simulink model "sensor_fusion_1"  (R2022b)
settings: Solver=FixedStepAuto  StartTime=0.0  StopTime=142  RelTol=1e-3  EnableMultiTasking=on
values from neighbouring files (symbols this model uses):
  A = [1.06559801427  0.0478097134081  -0.0142426631232; 0.0478097134081  0.959164863261  -0.0359507847494; -0.0142426631232  -0.0359507847494  0.982079248423]    [run1.mat]    (also in run1_wscan.mat; run2.mat; run2_wscan.mat; run3_wscan.mat)
  b = [2.14306210308 15.720848335 -0.863601368467]    [run1.mat]    (also in run1_wscan.mat; run2.mat; run2_wscan.mat; run3_wscan.mat)
  lut_in_model = [0.613658288305 4.0918386519 6.33532627088 8.02783554654 9.39128126795 10.3149653152 11.0684466084 11.9394591465 12.6234642167 13.2815233141 13.7919727262 14.1169774697 ... (18 elements, 1x18)]    [lut1.mat]    (also in lut2.mat = [2.20352000565 5.28649692724 7.42737645164 9.16368787483 10.; lut3.mat = [3.87191743285 4.36123645733 5.94318349981 7.0907146991 9.12; lut4.mat = [4.07430286502 6.74924870692 8.79421351968 10.2475792888 11.; run7_wscan.mat = [4.07430286502 6.74924870692 8.79421351968 10.2475792888 11.)
  lut_out_model = [4.36363636364 5.45454545455 6.54545454545 7.63636363636 8.72727272727 9.81818181818 10.9090909091 12 13.0909090909 14.1818181818 15.2727272727 16.3636363636 ... (18 elements, 1x18)]    [lut1.mat]    (also in lut2.mat; lut3.mat = [4.14545454545 4.36363636364 4.90909090909 5.45454545455 6.5; lut4.mat; run7_wscan.mat)
undefined symbols (not defined in the file or in its folder): ODR
libraries: raspberrypiBasiclib x6, simulink x4, raspberrypiIMUsensorslib x2, robotmobilelib x1, dspsigops x1
settings Model: Creator=sjohnson  LastModifiedBy=sjohnson
settings SolverCC: PositivePriorityOrder=on
settings OptimizationCC: EnhancedBackFolding=on  PassReuseOutputArgsAs=Individual arguments  ZeroExternalMemoryAtStartup=off  ZeroInternalMemoryAtStartup=off  MaxStackSize=64  OptimizeBlockOrder=speed  DifferentSizesBufferReuse=on  OptimizationCustomize=off  EfficientTunableParamExpr=on
settings DebuggingCC: ParameterTunabilityLossMsg=error
settings HardwareCC: ProdBitPerPointer=32  ProdBitPerSizeT=32  ProdBitPerPtrDiffT=32  ProdLargestAtomicInteger=Long  ProdLargestAtomicFloat=Double  ProdWordSize=32  ProdLongLongMode=on  ProdHWDeviceType=ARM Compatible->ARM Cortex  UseEmbeddedCoderFeatures=off  UseSimulinkCoderFeatures=off
settings RTWCC: Description=Embedded Coder  SystemTargetFile=ert.tlc  HardwareBoard=Raspberry Pi  TLCOptions="-aInlineSetEventsForThisBaseRateFcn=TLC_FALSE -aSuppressMultiTaskScheduler=TLC_FALSE  -aRateBasedStepFcn=0"  TemplateMakefile=ert_default_tmf  Toolchain=GNU GCC Embedded Linux  BuildConfiguration=Faster Runs
settings CodeAppCC: ForceParamTrailComments=on  IgnoreCustomStorageClasses=off  OperatorAnnotations=on  SimulinkDataObjDesc=on  SFDataObjDesc=on  InsertBlockDesc=on
settings ERTTargetCC: SupportNonInlinedSFcns=on  SupportVariableSizeSignals=on  ExtModeTransport=2  ExtModeStaticAlloc=on  ExtModeMexFile=ext_xcp  ExtModeIntrfLevel=Level2 - Open

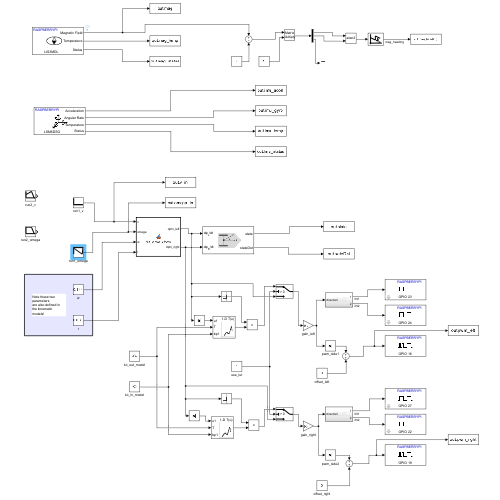
[thumbnail: Simulink's stored preview of the top-level diagram]
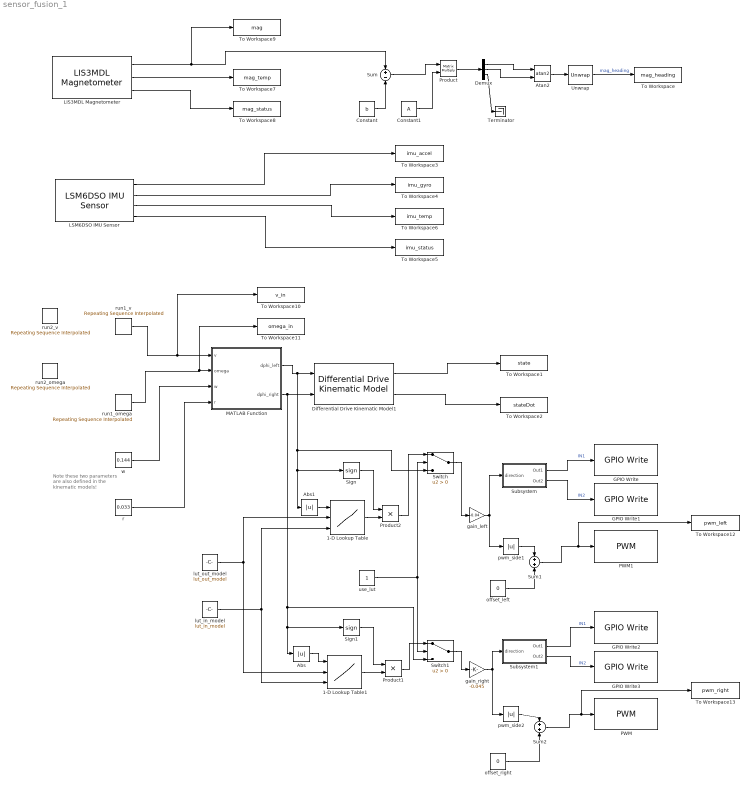
== system sensor_fusion_1 ==
  note: Note these two parameters
      | are also defined in the kinematic
      | models!
  1-D Lookup Table : Lookup_n-D  NumberOfTableDimensions=1  BreakpointsForDimension1Source=Input port  BreakpointsForDimension1=[-5:5]  IndexSearchMethod=Linear search  TableSource=Input port  Table=tanh([-5:5])  InterpMethod=Cubic spline  InternalRulePriority=Speed  RndMeth=Simplest
      settings: InputPortMap=u0,p221,p5
  1-D Lookup Table1 : Lookup_n-D  NumberOfTableDimensions=1  BreakpointsForDimension1Source=Input port  BreakpointsForDimension1=[-5:5]  IndexSearchMethod=Linear search  TableSource=Input port  Table=tanh([-5:5])  InterpMethod=Cubic spline  InternalRulePriority=Speed  RndMeth=Simplest
      settings: InputPortMap=u0,p221,p5
  Abs : Abs  SaturateOnIntegerOverflow=off
  Abs1 : Abs  SaturateOnIntegerOverflow=off
  Atan2 : Trigonometry  Operator=atan2
  Constant : Constant  Value=b
  Constant1 : Constant  Value=A
  Demux : Demux  Outputs=3
  Differential Drive Kinematic Model1 : robotmobilelib/Differential Drive Kinematic Model  VehicleInputs=Wheel Speeds  WheelRadius=.033  WheelSpeedRange=[-inf inf]  TrackWidth=0.144  InitialState=[0; 0; 0]  SimulateUsing=Interpreted execution
  GPIO Write : raspberrypiBasiclib/GPIO Write  board=Pi 4 Model B  gpio=23  direction=Output  blockPlatform=Raspberry Pi
  GPIO Write1 : raspberrypiBasiclib/GPIO Write  board=Pi 4 Model B  gpio=24  direction=Output  blockPlatform=Raspberry Pi
  GPIO Write2 : raspberrypiBasiclib/GPIO Write  board=Pi 4 Model B  gpio=27  direction=Output  blockPlatform=Raspberry Pi
  GPIO Write3 : raspberrypiBasiclib/GPIO Write  board=Pi 4 Model B  gpio=22  direction=Output  blockPlatform=Raspberry Pi
  LIS3MDL Magnetometer : raspberrypiIMUsensorslib/LIS3MDL Magnetometer  I2CModule=1  I2CAddress=0x1E  IsActiveMagnetometer=on  IsActiveTemperature=on  IsStatus=on  SampleTime=-1  MagnetometerRange=+/- 400 uT  MagnetometerODR=40 Hz
  LSM6DSO IMU Sensor : raspberrypiIMUsensorslib/LSM6DSO IMU Sensor  I2CModule=1  I2CAddress=0x6B  IsActiveAcceleration=on  IsActiveAngularRate=on  IsActiveTemperature=on  IsActiveStatus=on  IsActiveTimeStamp=off  SampleTime=-1  QueueSizeFactor=3  AccelerometerRange=+/- 2g  AccelerometerODR=52 Hz  AccelSelectCompositeFilter=No filter  AccelLPF2BW=ODR/4  AccelHPFBW=ODR/4  GyroscopeRange=1000 dps  GyroscopeODR=52 Hz  EnableGyroHPF=off  GyroHPFBW=0.016 Hz  EnableGyroLPF=off  GyroLPFBWMode=0
  MATLAB Function : MATLAB Function  TreatAsAtomicUnit=on
  PWM : raspberrypiBasiclib/PWM  board=Pi 4 Model B  Pin_=19  Frequency=40  blockPlatform=Raspberry Pi
  PWM1 : raspberrypiBasiclib/PWM  board=Pi 4 Model B  Pin_=18  Frequency=40  blockPlatform=Raspberry Pi
  Product : Product  Multiplication=Matrix(*)
  Product1 : Product
  Product2 : Product
  Sign : Signum
  Sign1 : Signum
  Subsystem : Subsystem
  Subsystem1 : Subsystem
  Sum : Sum  Inputs=+-
  Sum1 : Sum
  Sum2 : Sum
  Switch : Switch  Criteria=u2 > Threshold  SaturateOnIntegerOverflow=off  InputSameDT=off
  Switch1 : Switch  Criteria=u2 > Threshold  SaturateOnIntegerOverflow=off  InputSameDT=off
  Terminator : Terminator
  To Workspace : ToWorkspace  VariableName=mag_heading  SaveFormat=Structure With Time  SampleTime=-1
  To Workspace1 : ToWorkspace  VariableName=state  SaveFormat=Structure With Time  SampleTime=-1
  To Workspace10 : ToWorkspace  VariableName=v_in  SaveFormat=Structure With Time  SampleTime=-1
  To Workspace11 : ToWorkspace  VariableName=omega_in  SaveFormat=Structure With Time  SampleTime=-1
  To Workspace12 : ToWorkspace  VariableName=pwm_left  SaveFormat=Structure With Time  SampleTime=-1
  To Workspace13 : ToWorkspace  VariableName=pwm_right  SaveFormat=Structure With Time  SampleTime=-1
  To Workspace2 : ToWorkspace  VariableName=stateDot  SaveFormat=Structure With Time  SampleTime=-1
  To Workspace3 : ToWorkspace  VariableName=imu_accel  SaveFormat=Structure With Time  SampleTime=-1
  To Workspace4 : ToWorkspace  VariableName=imu_gyro  SaveFormat=Structure With Time  SampleTime=-1
  To Workspace5 : ToWorkspace  VariableName=imu_status  SaveFormat=Structure With Time  SampleTime=-1
  To Workspace6 : ToWorkspace  VariableName=imu_temp  SaveFormat=Structure With Time  SampleTime=-1
  To Workspace7 : ToWorkspace  VariableName=mag_temp  SaveFormat=Structure With Time  SampleTime=-1
  To Workspace8 : ToWorkspace  VariableName=mag_status  SaveFormat=Structure With Time  SampleTime=-1
  To Workspace9 : ToWorkspace  VariableName=mag  SaveFormat=Structure With Time  SampleTime=-1
  Unwrap : dspsigops/Unwrap  tol=pi  InputProcessing=Columns as channels (frame based)  running=off
  gain_left : Gain  Gain=-0.04
  gain_right : Gain  Gain=-0.045
  lut_in_model : Constant  Value=lut_in_model
  lut_out_model : Constant  Value=lut_out_model
  offset_left : Constant  Value=0
  offset_right : Constant  Value=0
  pwm_side1 : Abs  SaturateOnIntegerOverflow=off
  pwm_side2 : Abs  SaturateOnIntegerOverflow=off
  r : Constant  Value=0.033
  run1_omega : simulink/Sources/Repeating Sequence Interpolated  OutValues=-[0.5 1.0 1.5 2.0 2.5 3 3.5 4 4.5 5 5.5 6 6.5 7 0 0]  TimeValues=[0:10:140 142]  LookUpMeth=Use Input Below  tsamp=0.01  OutMin=[]  OutMax=[]  OutDataTypeStr=double  OutputDataTypeScalingMode=double  OutDataType=fixdt(0,8)  OutScaling=2^-10
  run1_v : simulink/Sources/Repeating Sequence Interpolated  OutValues=[0 0 0 0 0 0 0 0 0 0 0 0 0 0 0 0 0 0 0 0 0 0 0 0 0]  TimeValues=[0:10:230 232]  LookUpMeth=Use Input Below  tsamp=0.01  OutMin=[]  OutMax=[]  OutDataTypeStr=double  OutputDataTypeScalingMode=double  OutDataType=fixdt(0,8)  OutScaling=2^-10
  run2_omega : simulink/Sources/Repeating Sequence Interpolated  OutValues=[1 1 1 0.0 0.0]  TimeValues=[0 5 10 15 17]  LookUpMeth=Use Input Below  tsamp=0.01  OutMin=[]  OutMax=[]  OutDataTypeStr=double  OutputDataTypeScalingMode=double  OutDataType=fixdt(0,8)  OutScaling=2^-10
  run2_v : simulink/Sources/Repeating Sequence Interpolated  OutValues=[0.2 0.3 0.4 0 0]  TimeValues=[0 5 10 15 17]  LookUpMeth=Use Input Below  tsamp=0.01  OutMin=[]  OutMax=[]  OutDataTypeStr=double  OutputDataTypeScalingMode=double  OutDataType=fixdt(0,8)  OutScaling=2^-10
  use_lut : Constant
  w : Constant  Value=0.144
  wires:
  Differential Drive Kinematic Model1/1 -> To Workspace1/1
  Unwrap/1 -> To Workspace/1  "mag_heading"
  offset_right/1 -> Sum2/2
  Sum1/1 -> To Workspace12/1, PWM1/1
  pwm_side1/1 -> Sum1/1
  Sum2/1 -> To Workspace13/1, PWM/1
  MATLAB Function/2(dphi_right) -> Switch1/3, Sign1/1, Abs/1, Differential Drive Kinematic Model1/2
  Demux/1 -> Atan2/1
  Subsystem1/1(Out1) -> GPIO Write2/1  "IN1"
  Sum/1 -> Product/1
  Subsystem/1(Out1) -> GPIO Write/1  "IN1"
  Subsystem1/2(Out2) -> GPIO Write3/1  "IN2"
  offset_left/1 -> Sum1/2
  LIS3MDL Magnetometer/1 -> To Workspace9/1, Sum/1
  w/1 -> MATLAB Function/3(w)
  gain_right/1 -> pwm_side2/1, Subsystem1/1(direction)
  Atan2/1 -> Unwrap/1
  Constant/1 -> Sum/2
  run1_omega/1 -> To Workspace11/1, MATLAB Function/2(omega)
  pwm_side2/1 -> Sum2/1
  r/1 -> MATLAB Function/4(r)
  Differential Drive Kinematic Model1/2 -> To Workspace2/1
  LIS3MDL Magnetometer/3 -> To Workspace8/1
  gain_left/1 -> pwm_side1/1, Subsystem/1(direction)
  Subsystem/2(Out2) -> GPIO Write1/1  "IN2"
  MATLAB Function/1(dphi_left) -> Switch/3, Sign/1, Abs1/1, Differential Drive Kinematic Model1/1
  Demux/2 -> Atan2/2
  LIS3MDL Magnetometer/2 -> To Workspace7/1
  Constant1/1 -> Product/2
  Product/1 -> Demux/1
  LSM6DSO IMU Sensor/1 -> To Workspace3/1
  LSM6DSO IMU Sensor/4 -> To Workspace5/1
  LSM6DSO IMU Sensor/2 -> To Workspace4/1
  LSM6DSO IMU Sensor/3 -> To Workspace6/1
  Demux/3 -> Terminator/1
  run1_v/1 -> To Workspace10/1, MATLAB Function/1(v)
  lut_in_model/1 -> 1-D Lookup Table1/3, 1-D Lookup Table/3
  lut_out_model/1 -> 1-D Lookup Table1/2, 1-D Lookup Table/2
  1-D Lookup Table1/1 -> Product1/2
  Abs/1 -> 1-D Lookup Table1/1
  Abs1/1 -> 1-D Lookup Table/1
  Product1/1 -> Switch1/1
  Sign1/1 -> Product1/1
  Product2/1 -> Switch/1
  Sign/1 -> Product2/1
  1-D Lookup Table/1 -> Product2/2
  use_lut/1 -> Switch1/2, Switch/2
  Switch/1 -> gain_left/1
  Switch1/1 -> gain_right/1

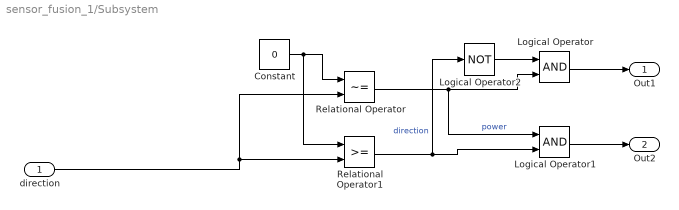
== system sensor_fusion_1/Subsystem ==
  direction : Inport
  Constant : Constant  Value=0
  Logical Operator : Logic  AllPortsSameDT=off  OutDataTypeStr=boolean
  Logical Operator1 : Logic  AllPortsSameDT=off  OutDataTypeStr=boolean
  Logical Operator2 : Logic  Operator=NOT  Inputs=1  AllPortsSameDT=off  OutDataTypeStr=boolean
  Relational Operator : RelationalOperator  Operator=~=  OutDataTypeStr=boolean  RndMeth=Simplest  InputSameDT=off
  Relational Operator1 : RelationalOperator  OutDataTypeStr=boolean  RndMeth=Simplest  InputSameDT=off
  Out1 : Outport
  Out2 : Outport  Port=2
  wires:
  Logical Operator/1 -> Out1/1
  Relational Operator1/1 -> Logical Operator2/1, Logical Operator1/2  "direction"
  Logical Operator1/1 -> Out2/1
  Logical Operator2/1 -> Logical Operator/1
  direction/1 -> Relational Operator/2, Relational Operator1/2
  Constant/1 -> Relational Operator1/1, Relational Operator/1
  Relational Operator/1 -> Logical Operator1/1, Logical Operator/2  "power"

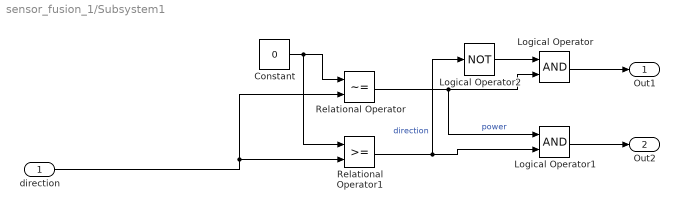
== system sensor_fusion_1/Subsystem1 ==
  direction : Inport
  Constant : Constant  Value=0
  Logical Operator : Logic  AllPortsSameDT=off  OutDataTypeStr=boolean
  Logical Operator1 : Logic  AllPortsSameDT=off  OutDataTypeStr=boolean
  Logical Operator2 : Logic  Operator=NOT  Inputs=1  AllPortsSameDT=off  OutDataTypeStr=boolean
  Relational Operator : RelationalOperator  Operator=~=  OutDataTypeStr=boolean  RndMeth=Simplest  InputSameDT=off
  Relational Operator1 : RelationalOperator  OutDataTypeStr=boolean  RndMeth=Simplest  InputSameDT=off
  Out1 : Outport
  Out2 : Outport  Port=2
  wires:
  Logical Operator/1 -> Out1/1
  Relational Operator1/1 -> Logical Operator2/1, Logical Operator1/2  "direction"
  Logical Operator1/1 -> Out2/1
  Logical Operator2/1 -> Logical Operator/1
  direction/1 -> Relational Operator/2, Relational Operator1/2
  Constant/1 -> Relational Operator1/1, Relational Operator/1
  Relational Operator/1 -> Logical Operator1/1, Logical Operator/2  "power"

== matlab function sensor_fusion_1/MATLAB Function ==
  data: v input; dphi_left output; omega input; w input; r input; dphi_right output
function [dphi_left, dphi_right] = diff_drive_xform(v, omega, w, r)

c1 = w/(2*r);
c2 = 2/w;

dphi_left = c1 * ( c2*v - omega );
dphi_right = c1 * ( c2*v + omega );
